simulink model "multiple_models_replacement"  (R2016a)
settings: Solver=VariableStepAuto  StartTime=0.0  StopTime=10.0  RelTol=1e-3
undefined symbols (not defined in the file): a2, b, b1, b2, eta, freq, g, J1, Jm1, Jw, Kem, kem, Kix, Kiy, Kpphi, Kpx, Kpy, kt, Kti, Kvphi, L, M, mi, mic, mis, N, R, r1, sigma0, sigma1, sigma2, Vdi, vs
settings Model: MinMaxOverflowLogging=ForceOff  sldv_blockreplacement_configurable_lib=multiple_models_rt_lib  Creator=Pichau  LastModifiedBy=Pichau
settings DataIOCC: SaveFormat=StructureWithTime  SaveOutput=off  SaveTime=off
settings DebuggingCC: ArtificialAlgebraicLoopMsg=none  SaveWithParameterizedLinksMsg=none  InheritedTsInSrcMsg=none  BusObjectLabelMismatch=none

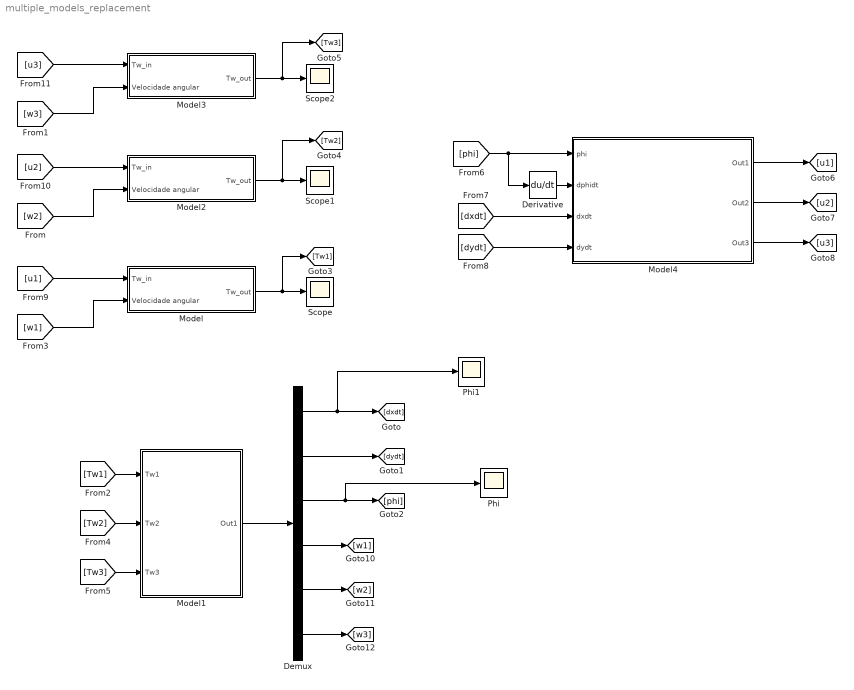
== system multiple_models_replacement ==
  Demux : Demux  Outputs=6
  Derivative : Derivative
  Model : Subsystem  TreatAsAtomicUnit=on  mask(Sldv ModelReference(Model name:modelo_eletrico) Replacement){ModelName=modelo_eletrico, ParameterArgumentNames=, ParameterArgumentValues=, SimulationMode=Normal}
      mask help: Replacement for the Model Reference block that references the model modelo_eletrico. If Model arguments are specified on the Model Reference block, then they will appear in the mask parameters.
  Model1 : Subsystem  TreatAsAtomicUnit=on  mask(Sldv ModelReference(Model name:modelo_mecanico) Replacement){ModelName=modelo_mecanico, ParameterArgumentNames=, ParameterArgumentValues=, SimulationMode=Normal}
      mask help: Replacement for the Model Reference block that references the model modelo_mecanico. If Model arguments are specified on the Model Reference block, then they will appear in the mask parameters.
  Model2 : Subsystem  TreatAsAtomicUnit=on  mask(Sldv ModelReference(Model name:modelo_eletrico) Replacement){ModelName=modelo_eletrico, ParameterArgumentNames=, ParameterArgumentValues=, SimulationMode=Normal}
      mask help: Replacement for the Model Reference block that references the model modelo_eletrico. If Model arguments are specified on the Model Reference block, then they will appear in the mask parameters.
  Model3 : Subsystem  TreatAsAtomicUnit=on  mask(Sldv ModelReference(Model name:modelo_eletrico) Replacement){ModelName=modelo_eletrico, ParameterArgumentNames=, ParameterArgumentValues=, SimulationMode=Normal}
      mask help: Replacement for the Model Reference block that references the model modelo_eletrico. If Model arguments are specified on the Model Reference block, then they will appear in the mask parameters.
  Model4 : Subsystem  TreatAsAtomicUnit=on  mask(Sldv ModelReference(Model name:resolved_acceleration_controller) Replacement){ModelName=resolved_acceleration_controller, ParameterArgumentNames=, ParameterArgumentValues=, SimulationMode=Normal}
      mask help: Replacement for the Model Reference block that references the model resolved_acceleration_controller. If Model arguments are specified on the Model Reference block, then they will appear in the mask parameters.
  Phi : Scope
  Phi1 : Scope
  Scope : Scope
  Scope1 : Scope
  Scope2 : Scope
  wires:
  [u1] -> Model/1(Tw_in)
  Model/1(Tw_out) -> [Tw1], Scope/1
  Model1/1(Out1) -> Demux/1
  Demux/3 -> Phi/1, [phi]
  Demux/4 -> [w1]
  Demux/5 -> [w2]
  Demux/6 -> [w3]
  Demux/1 -> Phi1/1, [dxdt]
  Demux/2 -> [dydt]
  [w1] -> Model/2(Velocidade angular)
  [u2] -> Model2/1(Tw_in)
  [w2] -> Model2/2(Velocidade angular)
  [u3] -> Model3/1(Tw_in)
  [w3] -> Model3/2(Velocidade angular)
  Model2/1(Tw_out) -> [Tw2], Scope1/1
  Model3/1(Tw_out) -> [Tw3], Scope2/1
  [Tw1] -> Model1/1(Tw1)
  [Tw3] -> Model1/3(Tw3)
  [Tw2] -> Model1/2(Tw2)
  Derivative/1 -> Model4/2(dphidt)
  [phi] -> Derivative/1, Model4/1(phi)
  [dxdt] -> Model4/3(dxdt)
  [dydt] -> Model4/4(dydt)
  Model4/1(Out1) -> [u1]
  Model4/2(Out2) -> [u2]
  Model4/3(Out3) -> [u3]

== system multiple_models_replacement/Model ==
  Tw_in : Inport  OutDataTypeStr=double  PortDimensions=1  SampleTime=[0,0]
  Velocidade angular : Inport  Port=2  OutDataTypeStr=double  PortDimensions=1  SampleTime=[0,0]
  1/r1 : Gain  Gain=r1
  1/r2 : Gain  Gain=r1
  Constant : Constant  Value=6
  Constant1 : Constant  Value=0.3
  Constant2 : Constant  Value=0
  Constant3 : Constant  Value=0
  Convergir torque para pulso : Subsystem
  Derivative : Derivative
  Roda1 : Subsystem
  dydt1 : Scope
  Tw_out : Outport  OutDataTypeStr=double  PortDimensions=1  SampleTime=[0,0]
  wires:
  Constant3/1 -> Roda1/6(s1)
  Constant2/1 -> Roda1/3(deltaVd1)
  Constant1/1 -> Roda1/1(Vsat1)
  Constant/1 -> Roda1/2(Vd1)
  1/r2/1 -> Tw_out/1
  Roda1/3(F1_aparente) -> 1/r2/1
  1/r1/1 -> Roda1/5(vel_lin1_aparente)
  [A] -> 1/r1/1
  Derivative/1 -> Convergir torque para pulso/2(aceleracao_angular)
  Velocidade angular/1 -> Derivative/1, [A], Convergir torque para pulso/3(velocidade angular)
  Tw_in/1 -> Convergir torque para pulso/1(Tw)
  Convergir torque para pulso/1(delta) -> dydt1/1, Roda1/4(u1)

== system multiple_models_replacement/Model1 ==
  Tw1 : Inport  OutDataTypeStr=double  PortDimensions=1  SampleTime=[0,0]
  Tw2 : Inport  Port=2  OutDataTypeStr=double  PortDimensions=1  SampleTime=[0,0]
  Tw3 : Inport  Port=3  OutDataTypeStr=double  PortDimensions=1  SampleTime=[0,0]
  Mux3 : Mux  Inputs=3
  Robô Omnidirecional : S-Function  FunctionName=espaco_de_estados  Parameters=r,m,Jw,J,L  SFunctionDeploymentMode=off  EnableBusSupport=off  mask{r=0.072, m=1.71, Jw=8.1e-4, J=2.125, L=0.09}
      mask prompts: r "r (m)"; m "m (Kg)"; Jw "Jw (Kg*m^2)"; J "J (Kg*m^2)"; L "L (m)"
      mask Display: image(imread('Robot_omnidirectional_drive.png'));
  Out1 : Outport  OutDataTypeStr=double  PortDimensions=6  SampleTime=[0,0]
  wires:
  Robô Omnidirecional/1 -> Out1/1
  Tw1/1 -> Mux3/1
  Tw2/1 -> Mux3/2
  Tw3/1 -> Mux3/3
  Mux3/1 -> Robô Omnidirecional/1

== system multiple_models_replacement/Model2 ==
  Tw_in : Inport  OutDataTypeStr=double  PortDimensions=1  SampleTime=[0,0]
  Velocidade angular : Inport  Port=2  OutDataTypeStr=double  PortDimensions=1  SampleTime=[0,0]
  1/r1 : Gain  Gain=r1
  1/r2 : Gain  Gain=r1
  Constant : Constant  Value=6
  Constant1 : Constant  Value=0.3
  Constant2 : Constant  Value=0
  Constant3 : Constant  Value=0
  Convergir torque para pulso : Subsystem
  Derivative : Derivative
  Roda1 : Subsystem
  dydt1 : Scope
  Tw_out : Outport  OutDataTypeStr=double  PortDimensions=1  SampleTime=[0,0]
  wires:
  Constant3/1 -> Roda1/6(s1)
  Constant2/1 -> Roda1/3(deltaVd1)
  Constant1/1 -> Roda1/1(Vsat1)
  Constant/1 -> Roda1/2(Vd1)
  1/r2/1 -> Tw_out/1
  Roda1/3(F1_aparente) -> 1/r2/1
  1/r1/1 -> Roda1/5(vel_lin1_aparente)
  [A] -> 1/r1/1
  Derivative/1 -> Convergir torque para pulso/2(aceleracao_angular)
  Velocidade angular/1 -> Derivative/1, [A], Convergir torque para pulso/3(velocidade angular)
  Tw_in/1 -> Convergir torque para pulso/1(Tw)
  Convergir torque para pulso/1(delta) -> dydt1/1, Roda1/4(u1)

== system multiple_models_replacement/Model3 ==
  Tw_in : Inport  OutDataTypeStr=double  PortDimensions=1  SampleTime=[0,0]
  Velocidade angular : Inport  Port=2  OutDataTypeStr=double  PortDimensions=1  SampleTime=[0,0]
  1/r1 : Gain  Gain=r1
  1/r2 : Gain  Gain=r1
  Constant : Constant  Value=6
  Constant1 : Constant  Value=0.3
  Constant2 : Constant  Value=0
  Constant3 : Constant  Value=0
  Convergir torque para pulso : Subsystem
  Derivative : Derivative
  Roda1 : Subsystem
  dydt1 : Scope
  Tw_out : Outport  OutDataTypeStr=double  PortDimensions=1  SampleTime=[0,0]
  wires:
  Constant3/1 -> Roda1/6(s1)
  Constant2/1 -> Roda1/3(deltaVd1)
  Constant1/1 -> Roda1/1(Vsat1)
  Constant/1 -> Roda1/2(Vd1)
  1/r2/1 -> Tw_out/1
  Roda1/3(F1_aparente) -> 1/r2/1
  1/r1/1 -> Roda1/5(vel_lin1_aparente)
  [A] -> 1/r1/1
  Derivative/1 -> Convergir torque para pulso/2(aceleracao_angular)
  Velocidade angular/1 -> Derivative/1, [A], Convergir torque para pulso/3(velocidade angular)
  Tw_in/1 -> Convergir torque para pulso/1(Tw)
  Convergir torque para pulso/1(delta) -> dydt1/1, Roda1/4(u1)

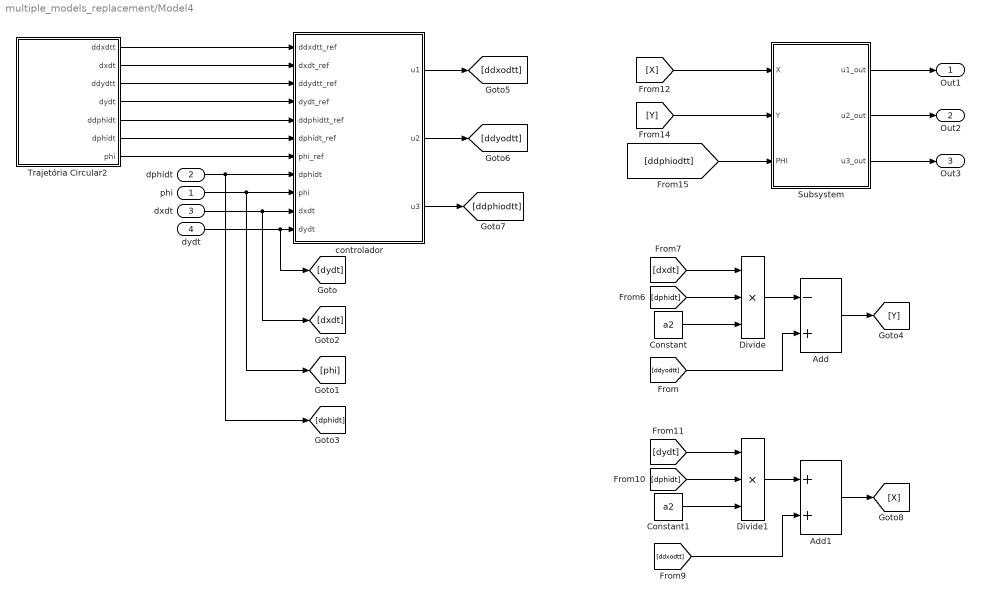
== system multiple_models_replacement/Model4 ==
  phi : Inport  OutDataTypeStr=double  PortDimensions=1  SampleTime=[0,0]
  dphidt : Inport  Port=2  OutDataTypeStr=double  PortDimensions=1  SampleTime=[0,0]
  dxdt : Inport  Port=3  OutDataTypeStr=double  PortDimensions=1  SampleTime=[0,0]
  dydt : Inport  Port=4  OutDataTypeStr=double  PortDimensions=1  SampleTime=[0,0]
  Add : Sum  Inputs=-+
  Add1 : Sum
  Constant : Constant  Value=a2
  Constant1 : Constant  Value=a2
  Divide : Product  Inputs=***
  Divide1 : Product  Inputs=***
  Subsystem : Subsystem
  Trajetória Circular2 : Subsystem
  controlador : Subsystem
  Out1 : Outport  OutDataTypeStr=double  PortDimensions=1  SampleTime=[0,0]
  Out2 : Outport  Port=2  OutDataTypeStr=double  PortDimensions=1  SampleTime=[0,0]
  Out3 : Outport  Port=3  OutDataTypeStr=double  PortDimensions=1  SampleTime=[0,0]
  wires:
  Subsystem/3(u3_out) -> Out3/1
  Subsystem/2(u2_out) -> Out2/1
  Subsystem/1(u1_out) -> Out1/1
  [ddphiodtt] -> Subsystem/3(PHI)
  [Y] -> Subsystem/2(Y)
  [X] -> Subsystem/1(X)
  Add1/1 -> [X]
  [ddxodtt] -> Add1/2
  Divide1/1 -> Add1/1
  [dydt] -> Divide1/1
  [dphidt] -> Divide1/2
  Constant1/1 -> Divide1/3
  Add/1 -> [Y]
  [ddyodtt] -> Add/2
  Divide/1 -> Add/1
  [dxdt] -> Divide/1
  [dphidt] -> Divide/2
  Constant/1 -> Divide/3
  dydt/1 -> [dydt], controlador/11(dydt)
  dxdt/1 -> [dxdt], controlador/10(dxdt)
  dphidt/1 -> [dphidt], controlador/8(dphidt)
  phi/1 -> [phi], controlador/9(phi)
  controlador/3(u3) -> [ddphiodtt]
  controlador/2(u2) -> [ddyodtt]
  controlador/1(u1) -> [ddxodtt]
  Trajetória Circular2/5(ddphidt) -> controlador/5(ddphidtt_ref)
  Trajetória Circular2/7(phi) -> controlador/7(phi_ref)
  Trajetória Circular2/3(ddydtt) -> controlador/3(ddydtt_ref)
  Trajetória Circular2/4(dydt) -> controlador/4(dydt_ref)
  Trajetória Circular2/1(ddxdtt) -> controlador/1(ddxdtt_ref)
  Trajetória Circular2/6(dphidt) -> controlador/6(dphidt_ref)
  Trajetória Circular2/2(dxdt) -> controlador/2(dxdt_ref)

== system multiple_models_replacement/Model/Convergir torque para pulso ==
  Tw : Inport
  aceleracao_angular : Inport  Port=2
  velocidade angular : Inport  Port=3
  Add : Sum  Inputs=+++
  Gain : Gain  Gain=R/(eta*N*Kti*Vdi)
  Gain1 : Gain  Gain=Kem
  Gain2 : Gain  Gain=R*Jw/(eta*N^2*Kti*Vdi)
  delta : Outport
  wires:
  aceleracao_angular/1 -> Gain2/1
  velocidade angular/1 -> Gain1/1
  Add/1 -> delta/1
  Tw/1 -> Gain/1
  Gain1/1 -> Add/3
  Gain/1 -> Add/1
  Gain2/1 -> Add/2

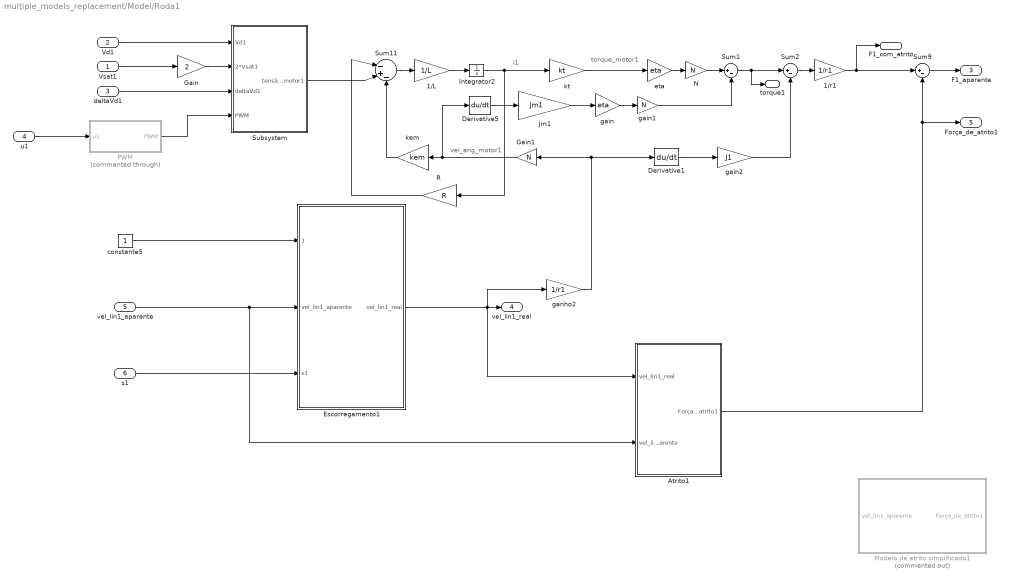
== system multiple_models_replacement/Model/Roda1 ==
  note: i1
  note: torque_motor1
  note: vel_ang_motor1
  Vsat1 : Inport
  Vd1 : Inport  Port=2
  deltaVd1 : Inport  Port=3
  u1 : Inport  Port=4
  vel_lin1_aparente : Inport  Port=5
  s1 : Inport  Port=6
  1/L : Gain  Gain=1/L
  1/r1 : Gain  Gain=1/r1
  Atrito1 : Subsystem
  Derivative1 : Derivative
  Derivative5 : Derivative
  Escorregamento1 : Subsystem
  Gain : Gain  Gain=2
  Gain1 : Gain  Gain=N
  Integrator2 : Integrator
  Jm1 : Gain  Gain=Jm1
  Modelo de atrito simplificado1 : Subsystem  Commented=on
  N : Gain  Gain=N
  PWM : Subsystem  Commented=through
  R : Gain  Gain=R
  Subsystem : Subsystem
  Sum1 : Sum  Inputs=|+-
  Sum11 : Sum  Inputs=|-+-
  Sum2 : Sum  Inputs=|+-
  Sum9 : Sum  Inputs=|+-
  constante5 : Constant
  eta : Gain  Gain=eta
  gain : Gain  Gain=eta
  gain1 : Gain  Gain=N
  gain2 : Gain  Gain=J1
  ganho2 : Gain  Gain=1/r1
  kem : Gain  Gain=kem
  kt : Gain  Gain=kt
  F1_com_atrito : Outport
  torque1 : Outport  Port=2
  F1_aparente : Outport  Port=3
  vel_lin1_real : Outport  Port=4
  Força_de_atrito1 : Outport  Port=5
  wires:
  Derivative5/1 -> Jm1/1
  Sum11/1 -> 1/L/1
  1/L/1 -> Integrator2/1
  Integrator2/1 -> kt/1, R/1
  Subsystem/1(tensão_motor1) -> Sum11/2
  kt/1 -> eta/1
  eta/1 -> N/1
  Gain1/1 -> kem/1, Derivative5/1
  1/r1/1 -> Sum9/1, F1_com_atrito/1
  Vsat1/1 -> Gain/1
  Vd1/1 -> Subsystem/1(Vd1)
  deltaVd1/1 -> Subsystem/3(deltaVd1)
  Gain/1 -> Subsystem/2("2*Vsat1 ")
  N/1 -> Sum1/1
  Sum1/1 -> torque1/1, Sum2/1
  gain/1 -> gain1/1
  Jm1/1 -> gain/1
  gain1/1 -> Sum1/2
  Derivative1/1 -> gain2/1
  gain2/1 -> Sum2/2
  Sum2/1 -> 1/r1/1
  kem/1 -> Sum11/3
  R/1 -> Sum11/1
  Sum9/1 -> F1_aparente/1
  u1/1 -> PWM/1(u1)
  Escorregamento1/1("vel_lin1_real ") -> Atrito1/1(vel_lin1_real), ganho2/1, vel_lin1_real/1
  ganho2/1 -> Derivative1/1, Gain1/1
  Atrito1/1(Força_de_atrito1) -> Sum9/2, Força_de_atrito1/1
  constante5/1 -> Escorregamento1/1(1)
  s1/1 -> Escorregamento1/3(s1)
  vel_lin1_aparente/1 -> Atrito1/2("vel_lin1_aparente "), Escorregamento1/2("vel_lin1_aparente ")
  PWM/1(PWM) -> Subsystem/4(PWM)

== system multiple_models_replacement/Model2/Convergir torque para pulso ==
  Tw : Inport
  aceleracao_angular : Inport  Port=2
  velocidade angular : Inport  Port=3
  Add : Sum  Inputs=+++
  Gain : Gain  Gain=R/(eta*N*Kti*Vdi)
  Gain1 : Gain  Gain=Kem
  Gain2 : Gain  Gain=R*Jw/(eta*N^2*Kti*Vdi)
  delta : Outport
  wires:
  aceleracao_angular/1 -> Gain2/1
  velocidade angular/1 -> Gain1/1
  Add/1 -> delta/1
  Tw/1 -> Gain/1
  Gain1/1 -> Add/3
  Gain/1 -> Add/1
  Gain2/1 -> Add/2

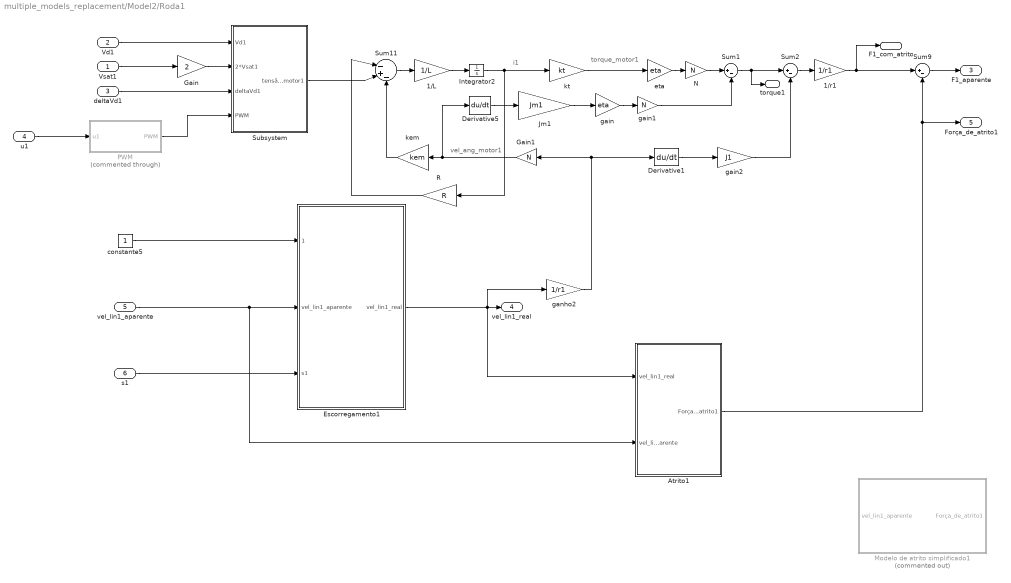
== system multiple_models_replacement/Model2/Roda1 ==
  note: i1
  note: torque_motor1
  note: vel_ang_motor1
  Vsat1 : Inport
  Vd1 : Inport  Port=2
  deltaVd1 : Inport  Port=3
  u1 : Inport  Port=4
  vel_lin1_aparente : Inport  Port=5
  s1 : Inport  Port=6
  1/L : Gain  Gain=1/L
  1/r1 : Gain  Gain=1/r1
  Atrito1 : Subsystem
  Derivative1 : Derivative
  Derivative5 : Derivative
  Escorregamento1 : Subsystem
  Gain : Gain  Gain=2
  Gain1 : Gain  Gain=N
  Integrator2 : Integrator
  Jm1 : Gain  Gain=Jm1
  Modelo de atrito simplificado1 : Subsystem  Commented=on
  N : Gain  Gain=N
  PWM : Subsystem  Commented=through
  R : Gain  Gain=R
  Subsystem : Subsystem
  Sum1 : Sum  Inputs=|+-
  Sum11 : Sum  Inputs=|-+-
  Sum2 : Sum  Inputs=|+-
  Sum9 : Sum  Inputs=|+-
  constante5 : Constant
  eta : Gain  Gain=eta
  gain : Gain  Gain=eta
  gain1 : Gain  Gain=N
  gain2 : Gain  Gain=J1
  ganho2 : Gain  Gain=1/r1
  kem : Gain  Gain=kem
  kt : Gain  Gain=kt
  F1_com_atrito : Outport
  torque1 : Outport  Port=2
  F1_aparente : Outport  Port=3
  vel_lin1_real : Outport  Port=4
  Força_de_atrito1 : Outport  Port=5
  wires:
  Derivative5/1 -> Jm1/1
  Sum11/1 -> 1/L/1
  1/L/1 -> Integrator2/1
  Integrator2/1 -> kt/1, R/1
  Subsystem/1(tensão_motor1) -> Sum11/2
  kt/1 -> eta/1
  eta/1 -> N/1
  Gain1/1 -> kem/1, Derivative5/1
  1/r1/1 -> Sum9/1, F1_com_atrito/1
  Vsat1/1 -> Gain/1
  Vd1/1 -> Subsystem/1(Vd1)
  deltaVd1/1 -> Subsystem/3(deltaVd1)
  Gain/1 -> Subsystem/2("2*Vsat1 ")
  N/1 -> Sum1/1
  Sum1/1 -> torque1/1, Sum2/1
  gain/1 -> gain1/1
  Jm1/1 -> gain/1
  gain1/1 -> Sum1/2
  Derivative1/1 -> gain2/1
  gain2/1 -> Sum2/2
  Sum2/1 -> 1/r1/1
  kem/1 -> Sum11/3
  R/1 -> Sum11/1
  Sum9/1 -> F1_aparente/1
  u1/1 -> PWM/1(u1)
  Escorregamento1/1("vel_lin1_real ") -> Atrito1/1(vel_lin1_real), ganho2/1, vel_lin1_real/1
  ganho2/1 -> Derivative1/1, Gain1/1
  Atrito1/1(Força_de_atrito1) -> Sum9/2, Força_de_atrito1/1
  constante5/1 -> Escorregamento1/1(1)
  s1/1 -> Escorregamento1/3(s1)
  vel_lin1_aparente/1 -> Atrito1/2("vel_lin1_aparente "), Escorregamento1/2("vel_lin1_aparente ")
  PWM/1(PWM) -> Subsystem/4(PWM)

== system multiple_models_replacement/Model3/Convergir torque para pulso ==
  Tw : Inport
  aceleracao_angular : Inport  Port=2
  velocidade angular : Inport  Port=3
  Add : Sum  Inputs=+++
  Gain : Gain  Gain=R/(eta*N*Kti*Vdi)
  Gain1 : Gain  Gain=Kem
  Gain2 : Gain  Gain=R*Jw/(eta*N^2*Kti*Vdi)
  delta : Outport
  wires:
  aceleracao_angular/1 -> Gain2/1
  velocidade angular/1 -> Gain1/1
  Add/1 -> delta/1
  Tw/1 -> Gain/1
  Gain1/1 -> Add/3
  Gain/1 -> Add/1
  Gain2/1 -> Add/2

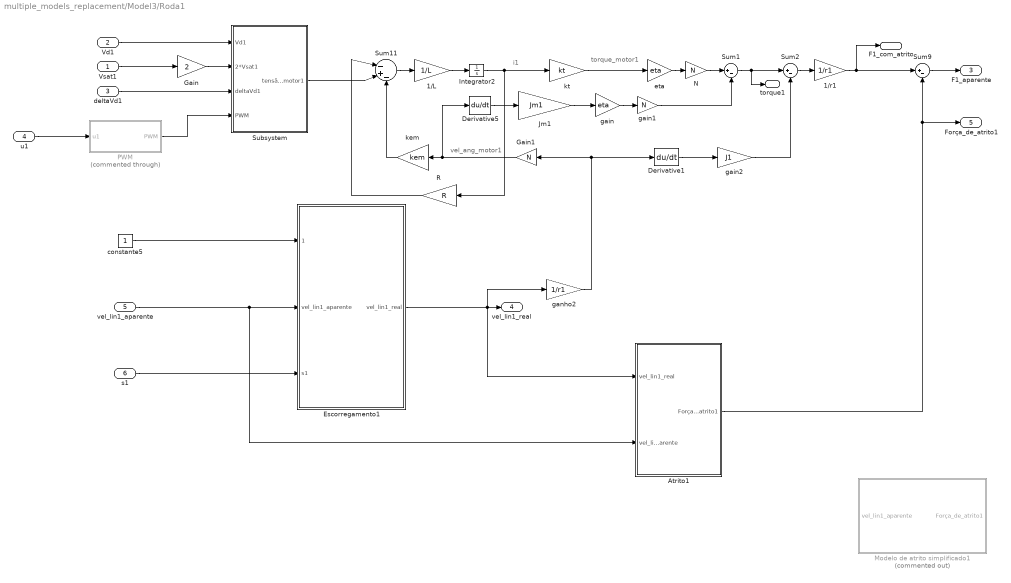
== system multiple_models_replacement/Model3/Roda1 ==
  note: i1
  note: torque_motor1
  note: vel_ang_motor1
  Vsat1 : Inport
  Vd1 : Inport  Port=2
  deltaVd1 : Inport  Port=3
  u1 : Inport  Port=4
  vel_lin1_aparente : Inport  Port=5
  s1 : Inport  Port=6
  1/L : Gain  Gain=1/L
  1/r1 : Gain  Gain=1/r1
  Atrito1 : Subsystem
  Derivative1 : Derivative
  Derivative5 : Derivative
  Escorregamento1 : Subsystem
  Gain : Gain  Gain=2
  Gain1 : Gain  Gain=N
  Integrator2 : Integrator
  Jm1 : Gain  Gain=Jm1
  Modelo de atrito simplificado1 : Subsystem  Commented=on
  N : Gain  Gain=N
  PWM : Subsystem  Commented=through
  R : Gain  Gain=R
  Subsystem : Subsystem
  Sum1 : Sum  Inputs=|+-
  Sum11 : Sum  Inputs=|-+-
  Sum2 : Sum  Inputs=|+-
  Sum9 : Sum  Inputs=|+-
  constante5 : Constant
  eta : Gain  Gain=eta
  gain : Gain  Gain=eta
  gain1 : Gain  Gain=N
  gain2 : Gain  Gain=J1
  ganho2 : Gain  Gain=1/r1
  kem : Gain  Gain=kem
  kt : Gain  Gain=kt
  F1_com_atrito : Outport
  torque1 : Outport  Port=2
  F1_aparente : Outport  Port=3
  vel_lin1_real : Outport  Port=4
  Força_de_atrito1 : Outport  Port=5
  wires:
  Derivative5/1 -> Jm1/1
  Sum11/1 -> 1/L/1
  1/L/1 -> Integrator2/1
  Integrator2/1 -> kt/1, R/1
  Subsystem/1(tensão_motor1) -> Sum11/2
  kt/1 -> eta/1
  eta/1 -> N/1
  Gain1/1 -> kem/1, Derivative5/1
  1/r1/1 -> Sum9/1, F1_com_atrito/1
  Vsat1/1 -> Gain/1
  Vd1/1 -> Subsystem/1(Vd1)
  deltaVd1/1 -> Subsystem/3(deltaVd1)
  Gain/1 -> Subsystem/2("2*Vsat1 ")
  N/1 -> Sum1/1
  Sum1/1 -> torque1/1, Sum2/1
  gain/1 -> gain1/1
  Jm1/1 -> gain/1
  gain1/1 -> Sum1/2
  Derivative1/1 -> gain2/1
  gain2/1 -> Sum2/2
  Sum2/1 -> 1/r1/1
  kem/1 -> Sum11/3
  R/1 -> Sum11/1
  Sum9/1 -> F1_aparente/1
  u1/1 -> PWM/1(u1)
  Escorregamento1/1("vel_lin1_real ") -> Atrito1/1(vel_lin1_real), ganho2/1, vel_lin1_real/1
  ganho2/1 -> Derivative1/1, Gain1/1
  Atrito1/1(Força_de_atrito1) -> Sum9/2, Força_de_atrito1/1
  constante5/1 -> Escorregamento1/1(1)
  s1/1 -> Escorregamento1/3(s1)
  vel_lin1_aparente/1 -> Atrito1/2("vel_lin1_aparente "), Escorregamento1/2("vel_lin1_aparente ")
  PWM/1(PWM) -> Subsystem/4(PWM)

== system multiple_models_replacement/Model4/Subsystem ==
  X : Inport
  Y : Inport  Port=2
  PHI : Inport  Port=3
  u1 : Subsystem
  u2 : Subsystem
  u3 : Subsystem
  u1_out : Outport
  u2_out : Outport  Port=2
  u3_out : Outport  Port=3
  wires:
  Y/1 -> u3/2(In2), u2/2(In2), u1/2(In2)
  PHI/1 -> u3/3(In3), u2/3(In3), u1/3(In3)
  X/1 -> u3/1(In1), u2/1(In1), u1/1(In1)
  u1/1(u1) -> u1_out/1
  u3/1(u3) -> u3_out/1
  u2/1(u2) -> u2_out/1

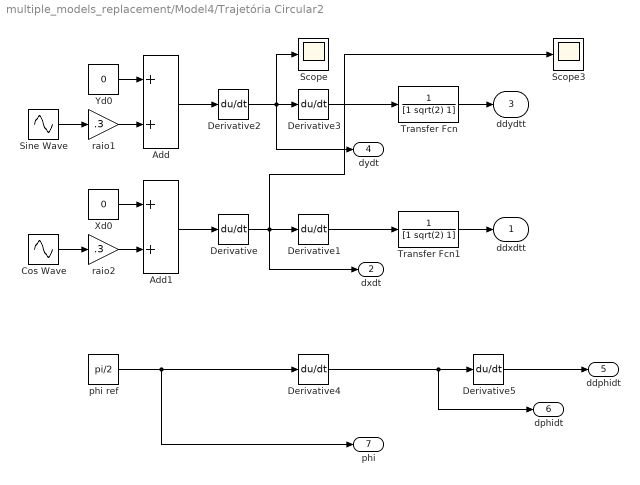
== system multiple_models_replacement/Model4/Trajetória Circular2 ==
  Add : Sum
  Add1 : Sum
  Cos Wave : Sin  Frequency=0.3  Phase=pi/2  SampleTime=0
  Derivative{,1..5} (6 alike) : Derivative
  Scope : Scope
  Scope3 : Scope
  Sine Wave : Sin  Frequency=0.3  SampleTime=0
  Transfer Fcn : TransferFcn  Denominator=[1 sqrt(2) 1]
  Transfer Fcn1 : TransferFcn  Denominator=[1 sqrt(2) 1]
  Xd0 : Constant  Value=0
  Yd0 : Constant  Value=0
  phi ref : Constant  Value=pi/2
  raio1 : Gain  Gain=.3
  raio2 : Gain  Gain=.3
  ddxdtt : Outport
  dxdt : Outport  Port=2
  ddydtt : Outport  Port=3
  dydt : Outport  Port=4
  ddphidt : Outport  Port=5
  dphidt : Outport  Port=6
  phi : Outport  Port=7
  wires:
  Transfer Fcn1/1 -> ddxdtt/1
  Transfer Fcn/1 -> ddydtt/1
  Derivative5/1 -> ddphidt/1
  Derivative1/1 -> Transfer Fcn1/1
  Derivative3/1 -> Transfer Fcn/1
  Derivative2/1 -> Derivative3/1, Scope/1, dydt/1
  Derivative/1 -> Scope3/1, Derivative1/1, dxdt/1
  Sine Wave/1 -> raio1/1
  raio1/1 -> Add/2
  Add/1 -> Derivative2/1
  Add1/1 -> Derivative/1
  raio2/1 -> Add1/2
  Cos Wave/1 -> raio2/1
  Xd0/1 -> Add1/1
  Yd0/1 -> Add/1
  phi ref/1 -> Derivative4/1, phi/1
  Derivative4/1 -> Derivative5/1, dphidt/1

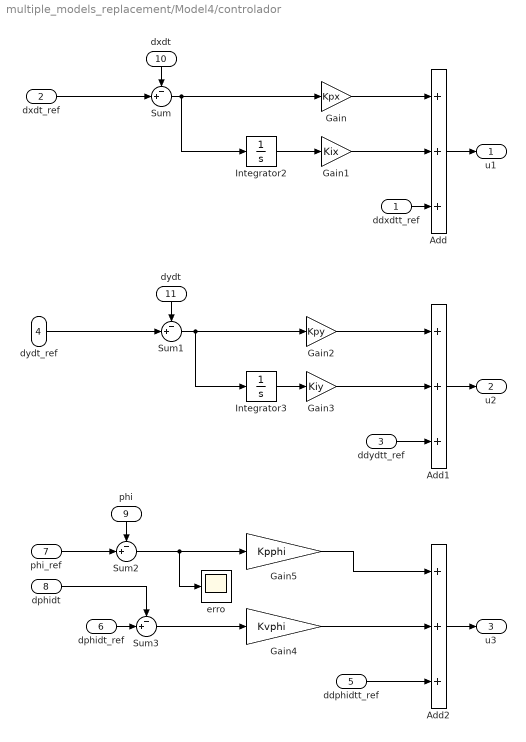
== system multiple_models_replacement/Model4/controlador ==
  ddxdtt_ref : Inport
  dxdt_ref : Inport  Port=2
  ddydtt_ref : Inport  Port=3
  dydt_ref : Inport  Port=4
  ddphidtt_ref : Inport  Port=5
  dphidt_ref : Inport  Port=6
  phi_ref : Inport  Port=7
  dphidt : Inport  Port=8
  phi : Inport  Port=9
  dxdt : Inport  Port=10
  dydt : Inport  Port=11
  Add : Sum  Inputs=+++
  Add1 : Sum  Inputs=+++
  Add2 : Sum  Inputs=+++
  Gain : Gain  Gain=Kpx
  Gain1 : Gain  Gain=Kix
  Gain2 : Gain  Gain=Kpy
  Gain3 : Gain  Gain=Kiy
  Gain4 : Gain  Gain=Kvphi
  Gain5 : Gain  Gain=Kpphi
  Integrator2 : Integrator
  Integrator3 : Integrator
  Sum{,1..3} (4 alike) : Sum  Inputs=-+|
  erro : Scope
  u1 : Outport
  u2 : Outport  Port=2
  u3 : Outport  Port=3
  wires:
  Sum2/1 -> Gain5/1, erro/1
  Sum1/1 -> Gain2/1, Integrator3/1
  Gain1/1 -> Add/2
  Integrator2/1 -> Gain1/1
  dydt_ref/1 -> Sum1/2
  Add/1 -> u1/1
  Gain2/1 -> Add1/1
  Integrator3/1 -> Gain3/1
  dphidt/1 -> Sum3/1
  Gain4/1 -> Add2/2
  Sum/1 -> Gain/1, Integrator2/1
  Gain3/1 -> Add1/2
  Gain5/1 -> Add2/1
  Sum3/1 -> Gain4/1
  ddphidtt_ref/1 -> Add2/3
  ddydtt_ref/1 -> Add1/3
  Add1/1 -> u2/1
  ddxdtt_ref/1 -> Add/3
  phi/1 -> Sum2/1
  Add2/1 -> u3/1
  dxdt_ref/1 -> Sum/2
  dxdt/1 -> Sum/1
  phi_ref/1 -> Sum2/2
  Gain/1 -> Add/1
  dydt/1 -> Sum1/1
  dphidt_ref/1 -> Sum3/2

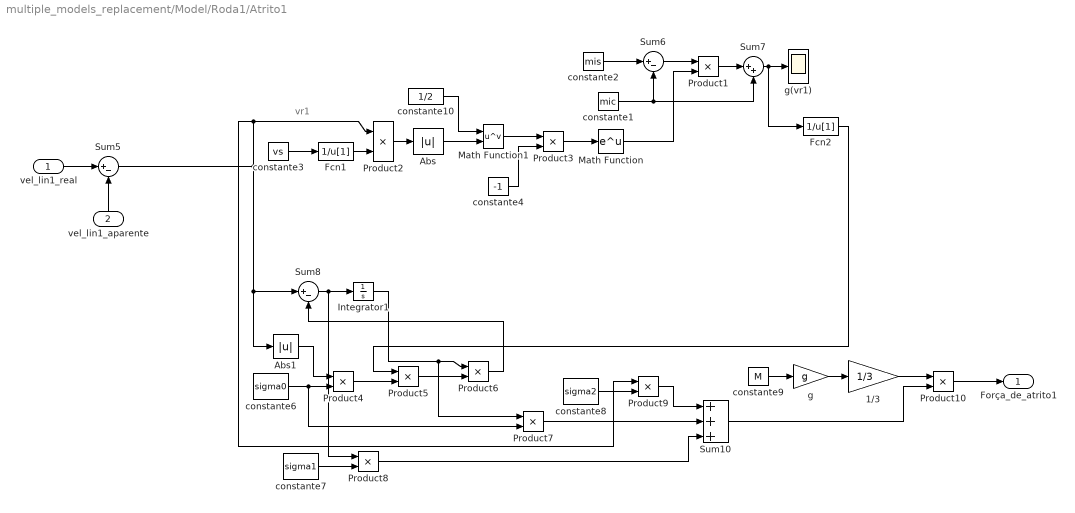
== system multiple_models_replacement/Model/Roda1/Atrito1 ==
  note: vr1
  vel_lin1_real : Inport
  "vel_lin1_aparente " : Inport  Port=2
  1/3 : Gain  Gain=1/3
  Abs : Abs
  Abs1 : Abs
  Fcn1 : Fcn  Expr=1/u[1]
  Fcn2 : Fcn  Expr=1/u[1]
  Integrator1 : Integrator
  Math Function : Math  SaturateOnIntegerOverflow=on
  Math Function1 : Math  Operator=pow  SaturateOnIntegerOverflow=on
  Product{1..10} (10 alike) : Product  RndMeth=Zero
  Sum10 : Sum  Inputs=+++
  Sum5 : Sum  Inputs=|+-
  Sum6 : Sum  Inputs=|+-
  Sum7 : Sum  Inputs=|++
  Sum8 : Sum  Inputs=|+-
  constante1 : Constant  Value=mic
  constante10 : Constant  Value=1/2
  constante2 : Constant  Value=mis
  constante3 : Constant  Value=vs
  constante4 : Constant  Value=-1
  constante6 : Constant  Value=sigma0
  constante7 : Constant  Value=sigma1
  constante8 : Constant  Value=sigma2
  constante9 : Constant  Value=M
  g : Gain  Gain=g
  g(vr1) : Scope
  Força_de_atrito1 : Outport
  wires:
  constante2/1 -> Sum6/1
  constante1/1 -> Sum6/2, Sum7/2
  Sum6/1 -> Product1/1
  constante3/1 -> Fcn1/1
  Fcn1/1 -> Product2/2
  Sum5/1 -> Sum8/1, Abs1/1, Product9/1, Product2/1
  Product2/1 -> Abs/1
  Abs/1 -> Math Function1/2
  Math Function1/1 -> Product3/1
  constante4/1 -> Product3/2
  Product3/1 -> Math Function/1
  Math Function/1 -> Product1/2
  Product1/1 -> Sum7/1
  Sum7/1 -> g(vr1)/1, Fcn2/1
  Sum8/1 -> Integrator1/1, Product8/1
  Integrator1/1 -> Product6/1, Product7/1
  constante6/1 -> Product4/2, Product7/2
  Abs1/1 -> Product4/1
  Product4/1 -> Product5/2
  Fcn2/1 -> Product5/1
  Product5/1 -> Product6/2
  Product6/1 -> Sum8/2
  constante7/1 -> Product8/2
  Product8/1 -> Sum10/3
  Product7/1 -> Sum10/2
  constante8/1 -> Product9/2
  Product9/1 -> Sum10/1
  constante9/1 -> g/1
  g/1 -> 1/3/1
  1/3/1 -> Product10/1
  Sum10/1 -> Product10/2
  constante10/1 -> Math Function1/1
  vel_lin1_real/1 -> Sum5/1
  "vel_lin1_aparente "/1 -> Sum5/2
  Product10/1 -> Força_de_atrito1/1

== system multiple_models_replacement/Model/Roda1/Escorregamento1 ==
  1 : Inport
  "vel_lin1_aparente " : Inport  Port=2
  s1 : Inport  Port=3
  Fcn : Fcn  Expr=1/u[1]
  Product : Product  RndMeth=Zero
  Sum3 : Sum  Inputs=+|+
  Sum4 : Sum  Inputs=|+-
  Switch : Switch
  "vel_lin1_real " : Outport
  wires:
  s1/1 -> Switch/2, Sum3/1, Sum4/2
  1/1 -> Sum3/2, Sum4/1
  Sum4/1 -> Fcn/1
  Fcn/1 -> Switch/1
  Sum3/1 -> Switch/3
  Switch/1 -> Product/2
  "vel_lin1_aparente "/1 -> Product/1
  Product/1 -> "vel_lin1_real "/1

== system multiple_models_replacement/Model/Roda1/Modelo de atrito simplificado1 ==
  vel_lin1_aparente : Inport
  1/3 : Gain  Gain=1/3
  Product10 : Product  RndMeth=Zero
  Scope : Scope
  Scope1 : Scope
  Scope2 : Scope
  Sign : Signum
  Sum1 : Sum  Inputs=++|
  Transfer Fcn : TransferFcn  Denominator=[0.001 1]
  constante9 : Constant  Value=M
  g : Gain  Gain=g
  g1 : Gain  Gain=mi
  g2 : Gain  Gain=b
  Força_de_atrito1 : Outport
  wires:
  Transfer Fcn/1 -> Força_de_atrito1/1, Scope2/1
  g2/1 -> Scope/1, Sum1/1
  Sum1/1 -> Transfer Fcn/1
  Sign/1 -> g1/1
  vel_lin1_aparente/1 -> Sign/1, g2/1
  Product10/1 -> Sum1/2, Scope1/1
  g1/1 -> Product10/2
  1/3/1 -> Product10/1
  g/1 -> 1/3/1
  constante9/1 -> g/1

== system multiple_models_replacement/Model/Roda1/PWM ==
  u1 : Inport
  Comparador : RelationalOperator  OutDataTypeStr=boolean
  Constant : Constant  Value=2
  Fcn : Fcn  Expr=2*(u(1)-0.5)
  Fcn1 : Fcn  Expr=2*((2*u[1]*freq)-0.5)
  Fcn2 : Fcn  Expr=u(1)-1
  Integrator : Integrator
  Onda Quadrada : Scope
  Onda Trinangular : Scope
  Product : Product  RndMeth=Zero
  Pulse Generator : DiscretePulseGenerator  PulseType=Time based  Period=1/freq  PulseWidth=50
  PWM : Outport
  wires:
  Pulse Generator/1 -> Fcn/1, Onda Quadrada/1
  Fcn/1 -> Integrator/1
  Integrator/1 -> Fcn1/1
  Fcn1/1 -> Onda Trinangular/1, Comparador/2
  u1/1 -> Comparador/1
  Fcn2/1 -> PWM/1
  Comparador/1 -> Product/2
  Product/1 -> Fcn2/1
  Constant/1 -> Product/1

== system multiple_models_replacement/Model/Roda1/Subsystem ==
  Vd1 : Inport
  "2*Vsat1 " : Inport  Port=2
  deltaVd1 : Inport  Port=3
  PWM : Inport  Port=4
  Product : Product  RndMeth=Zero
  Sum : Sum  Inputs=|+--
  tensão_motor1 : Outport
  wires:
  Sum/1 -> Product/1
  Vd1/1 -> Sum/1
  Product/1 -> tensão_motor1/1
  PWM/1 -> Product/2
  deltaVd1/1 -> Sum/3
  "2*Vsat1 "/1 -> Sum/2

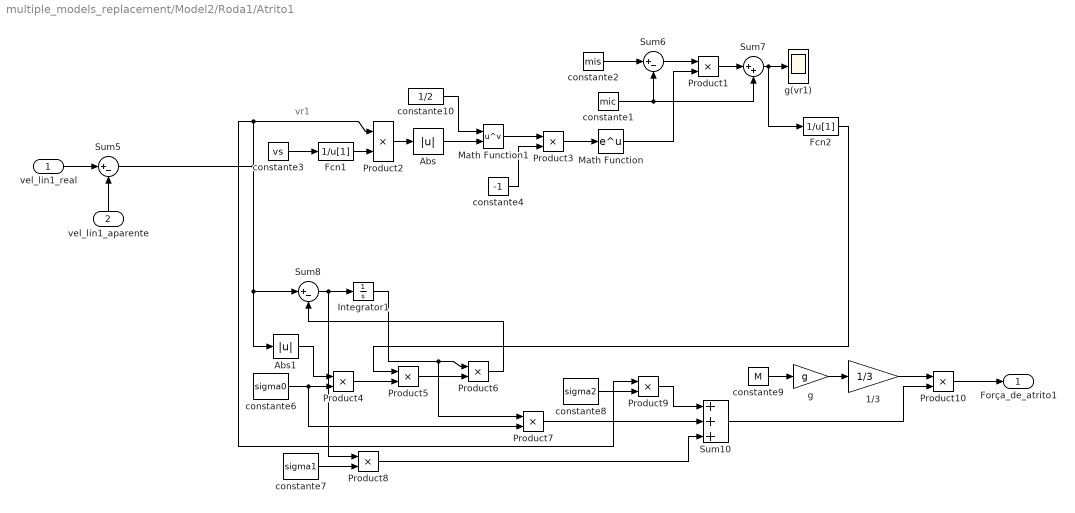
== system multiple_models_replacement/Model2/Roda1/Atrito1 ==
  note: vr1
  vel_lin1_real : Inport
  "vel_lin1_aparente " : Inport  Port=2
  1/3 : Gain  Gain=1/3
  Abs : Abs
  Abs1 : Abs
  Fcn1 : Fcn  Expr=1/u[1]
  Fcn2 : Fcn  Expr=1/u[1]
  Integrator1 : Integrator
  Math Function : Math  SaturateOnIntegerOverflow=on
  Math Function1 : Math  Operator=pow  SaturateOnIntegerOverflow=on
  Product{1..10} (10 alike) : Product  RndMeth=Zero
  Sum10 : Sum  Inputs=+++
  Sum5 : Sum  Inputs=|+-
  Sum6 : Sum  Inputs=|+-
  Sum7 : Sum  Inputs=|++
  Sum8 : Sum  Inputs=|+-
  constante1 : Constant  Value=mic
  constante10 : Constant  Value=1/2
  constante2 : Constant  Value=mis
  constante3 : Constant  Value=vs
  constante4 : Constant  Value=-1
  constante6 : Constant  Value=sigma0
  constante7 : Constant  Value=sigma1
  constante8 : Constant  Value=sigma2
  constante9 : Constant  Value=M
  g : Gain  Gain=g
  g(vr1) : Scope
  Força_de_atrito1 : Outport
  wires:
  constante2/1 -> Sum6/1
  constante1/1 -> Sum6/2, Sum7/2
  Sum6/1 -> Product1/1
  constante3/1 -> Fcn1/1
  Fcn1/1 -> Product2/2
  Sum5/1 -> Sum8/1, Abs1/1, Product9/1, Product2/1
  Product2/1 -> Abs/1
  Abs/1 -> Math Function1/2
  Math Function1/1 -> Product3/1
  constante4/1 -> Product3/2
  Product3/1 -> Math Function/1
  Math Function/1 -> Product1/2
  Product1/1 -> Sum7/1
  Sum7/1 -> g(vr1)/1, Fcn2/1
  Sum8/1 -> Integrator1/1, Product8/1
  Integrator1/1 -> Product6/1, Product7/1
  constante6/1 -> Product4/2, Product7/2
  Abs1/1 -> Product4/1
  Product4/1 -> Product5/2
  Fcn2/1 -> Product5/1
  Product5/1 -> Product6/2
  Product6/1 -> Sum8/2
  constante7/1 -> Product8/2
  Product8/1 -> Sum10/3
  Product7/1 -> Sum10/2
  constante8/1 -> Product9/2
  Product9/1 -> Sum10/1
  constante9/1 -> g/1
  g/1 -> 1/3/1
  1/3/1 -> Product10/1
  Sum10/1 -> Product10/2
  constante10/1 -> Math Function1/1
  vel_lin1_real/1 -> Sum5/1
  "vel_lin1_aparente "/1 -> Sum5/2
  Product10/1 -> Força_de_atrito1/1

== system multiple_models_replacement/Model2/Roda1/Escorregamento1 ==
  1 : Inport
  "vel_lin1_aparente " : Inport  Port=2
  s1 : Inport  Port=3
  Fcn : Fcn  Expr=1/u[1]
  Product : Product  RndMeth=Zero
  Sum3 : Sum  Inputs=+|+
  Sum4 : Sum  Inputs=|+-
  Switch : Switch
  "vel_lin1_real " : Outport
  wires:
  s1/1 -> Switch/2, Sum3/1, Sum4/2
  1/1 -> Sum3/2, Sum4/1
  Sum4/1 -> Fcn/1
  Fcn/1 -> Switch/1
  Sum3/1 -> Switch/3
  Switch/1 -> Product/2
  "vel_lin1_aparente "/1 -> Product/1
  Product/1 -> "vel_lin1_real "/1

== system multiple_models_replacement/Model2/Roda1/Modelo de atrito simplificado1 ==
  vel_lin1_aparente : Inport
  1/3 : Gain  Gain=1/3
  Product10 : Product  RndMeth=Zero
  Scope : Scope
  Scope1 : Scope
  Scope2 : Scope
  Sign : Signum
  Sum1 : Sum  Inputs=++|
  Transfer Fcn : TransferFcn  Denominator=[0.001 1]
  constante9 : Constant  Value=M
  g : Gain  Gain=g
  g1 : Gain  Gain=mi
  g2 : Gain  Gain=b
  Força_de_atrito1 : Outport
  wires:
  Transfer Fcn/1 -> Força_de_atrito1/1, Scope2/1
  g2/1 -> Scope/1, Sum1/1
  Sum1/1 -> Transfer Fcn/1
  Sign/1 -> g1/1
  vel_lin1_aparente/1 -> Sign/1, g2/1
  Product10/1 -> Sum1/2, Scope1/1
  g1/1 -> Product10/2
  1/3/1 -> Product10/1
  g/1 -> 1/3/1
  constante9/1 -> g/1

== system multiple_models_replacement/Model2/Roda1/PWM ==
  u1 : Inport
  Comparador : RelationalOperator  OutDataTypeStr=boolean
  Constant : Constant  Value=2
  Fcn : Fcn  Expr=2*(u(1)-0.5)
  Fcn1 : Fcn  Expr=2*((2*u[1]*freq)-0.5)
  Fcn2 : Fcn  Expr=u(1)-1
  Integrator : Integrator
  Onda Quadrada : Scope
  Onda Trinangular : Scope
  Product : Product  RndMeth=Zero
  Pulse Generator : DiscretePulseGenerator  PulseType=Time based  Period=1/freq  PulseWidth=50
  PWM : Outport
  wires:
  Pulse Generator/1 -> Fcn/1, Onda Quadrada/1
  Fcn/1 -> Integrator/1
  Integrator/1 -> Fcn1/1
  Fcn1/1 -> Onda Trinangular/1, Comparador/2
  u1/1 -> Comparador/1
  Fcn2/1 -> PWM/1
  Comparador/1 -> Product/2
  Product/1 -> Fcn2/1
  Constant/1 -> Product/1

== system multiple_models_replacement/Model2/Roda1/Subsystem ==
  Vd1 : Inport
  "2*Vsat1 " : Inport  Port=2
  deltaVd1 : Inport  Port=3
  PWM : Inport  Port=4
  Product : Product  RndMeth=Zero
  Sum : Sum  Inputs=|+--
  tensão_motor1 : Outport
  wires:
  Sum/1 -> Product/1
  Vd1/1 -> Sum/1
  Product/1 -> tensão_motor1/1
  PWM/1 -> Product/2
  deltaVd1/1 -> Sum/3
  "2*Vsat1 "/1 -> Sum/2

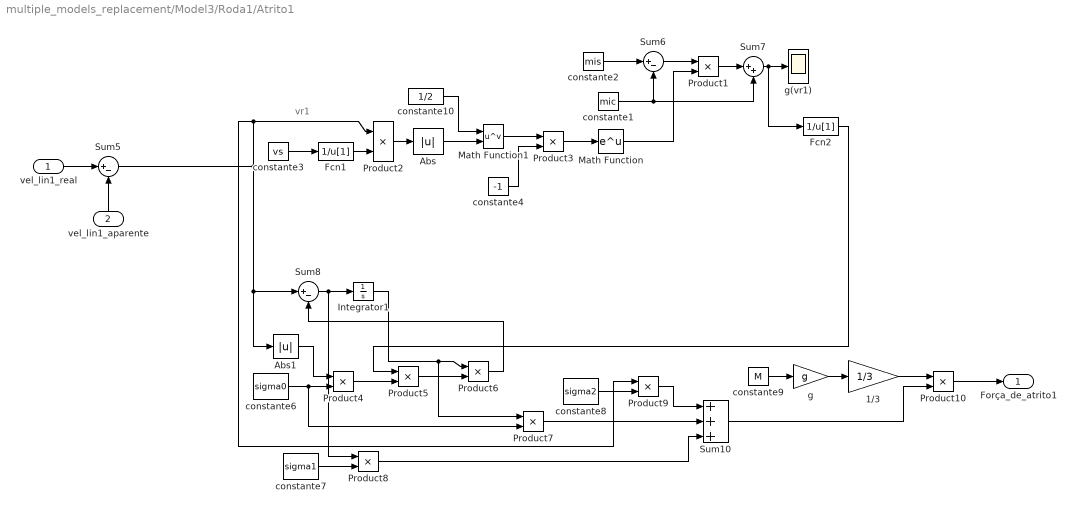
== system multiple_models_replacement/Model3/Roda1/Atrito1 ==
  note: vr1
  vel_lin1_real : Inport
  "vel_lin1_aparente " : Inport  Port=2
  1/3 : Gain  Gain=1/3
  Abs : Abs
  Abs1 : Abs
  Fcn1 : Fcn  Expr=1/u[1]
  Fcn2 : Fcn  Expr=1/u[1]
  Integrator1 : Integrator
  Math Function : Math  SaturateOnIntegerOverflow=on
  Math Function1 : Math  Operator=pow  SaturateOnIntegerOverflow=on
  Product{1..10} (10 alike) : Product  RndMeth=Zero
  Sum10 : Sum  Inputs=+++
  Sum5 : Sum  Inputs=|+-
  Sum6 : Sum  Inputs=|+-
  Sum7 : Sum  Inputs=|++
  Sum8 : Sum  Inputs=|+-
  constante1 : Constant  Value=mic
  constante10 : Constant  Value=1/2
  constante2 : Constant  Value=mis
  constante3 : Constant  Value=vs
  constante4 : Constant  Value=-1
  constante6 : Constant  Value=sigma0
  constante7 : Constant  Value=sigma1
  constante8 : Constant  Value=sigma2
  constante9 : Constant  Value=M
  g : Gain  Gain=g
  g(vr1) : Scope
  Força_de_atrito1 : Outport
  wires:
  constante2/1 -> Sum6/1
  constante1/1 -> Sum6/2, Sum7/2
  Sum6/1 -> Product1/1
  constante3/1 -> Fcn1/1
  Fcn1/1 -> Product2/2
  Sum5/1 -> Sum8/1, Abs1/1, Product9/1, Product2/1
  Product2/1 -> Abs/1
  Abs/1 -> Math Function1/2
  Math Function1/1 -> Product3/1
  constante4/1 -> Product3/2
  Product3/1 -> Math Function/1
  Math Function/1 -> Product1/2
  Product1/1 -> Sum7/1
  Sum7/1 -> g(vr1)/1, Fcn2/1
  Sum8/1 -> Integrator1/1, Product8/1
  Integrator1/1 -> Product6/1, Product7/1
  constante6/1 -> Product4/2, Product7/2
  Abs1/1 -> Product4/1
  Product4/1 -> Product5/2
  Fcn2/1 -> Product5/1
  Product5/1 -> Product6/2
  Product6/1 -> Sum8/2
  constante7/1 -> Product8/2
  Product8/1 -> Sum10/3
  Product7/1 -> Sum10/2
  constante8/1 -> Product9/2
  Product9/1 -> Sum10/1
  constante9/1 -> g/1
  g/1 -> 1/3/1
  1/3/1 -> Product10/1
  Sum10/1 -> Product10/2
  constante10/1 -> Math Function1/1
  vel_lin1_real/1 -> Sum5/1
  "vel_lin1_aparente "/1 -> Sum5/2
  Product10/1 -> Força_de_atrito1/1

== system multiple_models_replacement/Model3/Roda1/Escorregamento1 ==
  1 : Inport
  "vel_lin1_aparente " : Inport  Port=2
  s1 : Inport  Port=3
  Fcn : Fcn  Expr=1/u[1]
  Product : Product  RndMeth=Zero
  Sum3 : Sum  Inputs=+|+
  Sum4 : Sum  Inputs=|+-
  Switch : Switch
  "vel_lin1_real " : Outport
  wires:
  s1/1 -> Switch/2, Sum3/1, Sum4/2
  1/1 -> Sum3/2, Sum4/1
  Sum4/1 -> Fcn/1
  Fcn/1 -> Switch/1
  Sum3/1 -> Switch/3
  Switch/1 -> Product/2
  "vel_lin1_aparente "/1 -> Product/1
  Product/1 -> "vel_lin1_real "/1

== system multiple_models_replacement/Model3/Roda1/Modelo de atrito simplificado1 ==
  vel_lin1_aparente : Inport
  1/3 : Gain  Gain=1/3
  Product10 : Product  RndMeth=Zero
  Scope : Scope
  Scope1 : Scope
  Scope2 : Scope
  Sign : Signum
  Sum1 : Sum  Inputs=++|
  Transfer Fcn : TransferFcn  Denominator=[0.001 1]
  constante9 : Constant  Value=M
  g : Gain  Gain=g
  g1 : Gain  Gain=mi
  g2 : Gain  Gain=b
  Força_de_atrito1 : Outport
  wires:
  Transfer Fcn/1 -> Força_de_atrito1/1, Scope2/1
  g2/1 -> Scope/1, Sum1/1
  Sum1/1 -> Transfer Fcn/1
  Sign/1 -> g1/1
  vel_lin1_aparente/1 -> Sign/1, g2/1
  Product10/1 -> Sum1/2, Scope1/1
  g1/1 -> Product10/2
  1/3/1 -> Product10/1
  g/1 -> 1/3/1
  constante9/1 -> g/1

== system multiple_models_replacement/Model3/Roda1/PWM ==
  u1 : Inport
  Comparador : RelationalOperator  OutDataTypeStr=boolean
  Constant : Constant  Value=2
  Fcn : Fcn  Expr=2*(u(1)-0.5)
  Fcn1 : Fcn  Expr=2*((2*u[1]*freq)-0.5)
  Fcn2 : Fcn  Expr=u(1)-1
  Integrator : Integrator
  Onda Quadrada : Scope
  Onda Trinangular : Scope
  Product : Product  RndMeth=Zero
  Pulse Generator : DiscretePulseGenerator  PulseType=Time based  Period=1/freq  PulseWidth=50
  PWM : Outport
  wires:
  Pulse Generator/1 -> Fcn/1, Onda Quadrada/1
  Fcn/1 -> Integrator/1
  Integrator/1 -> Fcn1/1
  Fcn1/1 -> Onda Trinangular/1, Comparador/2
  u1/1 -> Comparador/1
  Fcn2/1 -> PWM/1
  Comparador/1 -> Product/2
  Product/1 -> Fcn2/1
  Constant/1 -> Product/1

== system multiple_models_replacement/Model3/Roda1/Subsystem ==
  Vd1 : Inport
  "2*Vsat1 " : Inport  Port=2
  deltaVd1 : Inport  Port=3
  PWM : Inport  Port=4
  Product : Product  RndMeth=Zero
  Sum : Sum  Inputs=|+--
  tensão_motor1 : Outport
  wires:
  Sum/1 -> Product/1
  Vd1/1 -> Sum/1
  Product/1 -> tensão_motor1/1
  PWM/1 -> Product/2
  deltaVd1/1 -> Sum/3
  "2*Vsat1 "/1 -> Sum/2

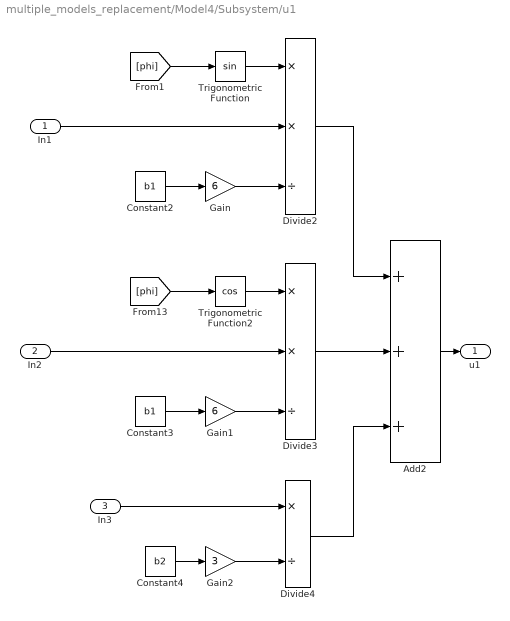
== system multiple_models_replacement/Model4/Subsystem/u1 ==
  In1 : Inport
  In2 : Inport  Port=2
  In3 : Inport  Port=3
  Add2 : Sum  Inputs=+++
  Constant2 : Constant  Value=b1
  Constant3 : Constant  Value=b1
  Constant4 : Constant  Value=b2
  Divide2 : Product  Inputs=**/
  Divide3 : Product  Inputs=**/
  Divide4 : Product  Inputs=*/
  Gain : Gain  Gain=6
  Gain1 : Gain  Gain=6
  Gain2 : Gain  Gain=3
  Trigonometric Function : Trigonometry
  Trigonometric Function2 : Trigonometry  Operator=cos
  u1 : Outport
  wires:
  Add2/1 -> u1/1
  Divide3/1 -> Add2/2
  Divide4/1 -> Add2/3
  In1/1 -> Divide2/2
  Gain2/1 -> Divide4/2
  Constant2/1 -> Gain/1
  Gain/1 -> Divide2/3
  [phi] -> Trigonometric Function/1
  Divide2/1 -> Add2/1
  Constant4/1 -> Gain2/1
  [phi] -> Trigonometric Function2/1
  Trigonometric Function2/1 -> Divide3/1
  In2/1 -> Divide3/2
  Constant3/1 -> Gain1/1
  Gain1/1 -> Divide3/3
  Trigonometric Function/1 -> Divide2/1
  In3/1 -> Divide4/1

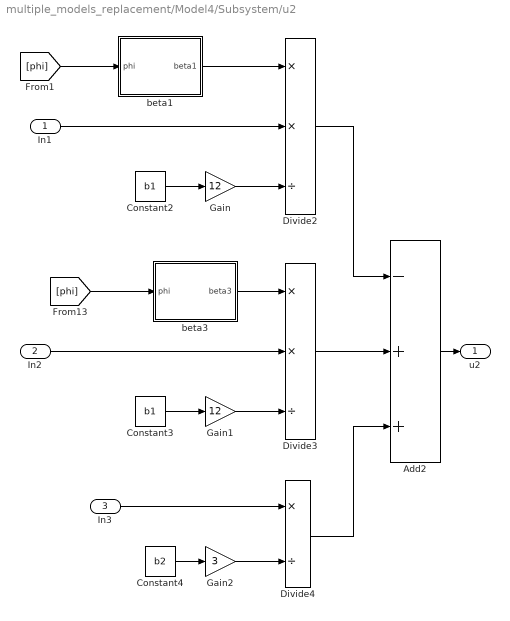
== system multiple_models_replacement/Model4/Subsystem/u2 ==
  In1 : Inport
  In2 : Inport  Port=2
  In3 : Inport  Port=3
  Add2 : Sum  Inputs=-++
  Constant2 : Constant  Value=b1
  Constant3 : Constant  Value=b1
  Constant4 : Constant  Value=b2
  Divide2 : Product  Inputs=**/
  Divide3 : Product  Inputs=**/
  Divide4 : Product  Inputs=*/
  Gain : Gain  Gain=12
  Gain1 : Gain  Gain=12
  Gain2 : Gain  Gain=3
  beta1 : Subsystem
  beta3 : Subsystem
  u2 : Outport
  wires:
  In3/1 -> Divide4/1
  beta1/1(beta1) -> Divide2/1
  Gain1/1 -> Divide3/3
  Constant3/1 -> Gain1/1
  In2/1 -> Divide3/2
  beta3/1(beta3) -> Divide3/1
  [phi] -> beta3/1(phi)
  Constant4/1 -> Gain2/1
  Divide2/1 -> Add2/1
  [phi] -> beta1/1(phi)
  Gain/1 -> Divide2/3
  Constant2/1 -> Gain/1
  Gain2/1 -> Divide4/2
  In1/1 -> Divide2/2
  Divide4/1 -> Add2/3
  Divide3/1 -> Add2/2
  Add2/1 -> u2/1

== system multiple_models_replacement/Model4/Subsystem/u3 ==
  In1 : Inport
  In2 : Inport  Port=2
  In3 : Inport  Port=3
  Add2 : Sum  Inputs=-++
  Constant2 : Constant  Value=b1
  Constant3 : Constant  Value=b1
  Constant4 : Constant  Value=b2
  Divide2 : Product  Inputs=**/
  Divide3 : Product  Inputs=**/
  Divide4 : Product  Inputs=*/
  Gain : Gain  Gain=12
  Gain1 : Gain  Gain=12
  Gain2 : Gain  Gain=3
  beta2 : Subsystem
  beta4 : Subsystem
  u3 : Outport
  wires:
  In3/1 -> Divide4/1
  beta2/1(beta2) -> Divide2/1
  Gain1/1 -> Divide3/3
  Constant3/1 -> Gain1/1
  In2/1 -> Divide3/2
  beta4/1(beta4) -> Divide3/1
  [phi] -> beta4/1(phi)
  Constant4/1 -> Gain2/1
  Divide2/1 -> Add2/1
  [phi] -> beta2/1(phi)
  Gain/1 -> Divide2/3
  Constant2/1 -> Gain/1
  Gain2/1 -> Divide4/2
  In1/1 -> Divide2/2
  Divide4/1 -> Add2/3
  Divide3/1 -> Add2/2
  Add2/1 -> u3/1

== system multiple_models_replacement/Model4/Subsystem/u2/beta1 ==
  phi : Inport
  Add2 : Sum  Inputs=+-
  Constant2 : Constant  Value=3
  Divide2 : Product  Inputs=**
  Sqrt : Sqrt  SaturateOnIntegerOverflow=on
  Trigonometric Function1 : Trigonometry  Operator=cos
  Trigonometric Function2 : Trigonometry
  beta1 : Outport
  wires:
  Trigonometric Function2/1 -> Add2/1
  phi/1 -> Trigonometric Function1/1, Trigonometric Function2/1
  Constant2/1 -> Sqrt/1
  Sqrt/1 -> Divide2/2
  Add2/1 -> beta1/1
  Trigonometric Function1/1 -> Divide2/1
  Divide2/1 -> Add2/2

== system multiple_models_replacement/Model4/Subsystem/u2/beta3 ==
  phi : Inport
  Add2 : Sum
  Constant2 : Constant  Value=3
  Divide2 : Product  Inputs=**
  Sqrt : Sqrt  SaturateOnIntegerOverflow=on
  Trigonometric Function1 : Trigonometry
  Trigonometric Function2 : Trigonometry  Operator=cos
  beta3 : Outport
  wires:
  Trigonometric Function2/1 -> Add2/1
  phi/1 -> Trigonometric Function1/1, Trigonometric Function2/1
  Constant2/1 -> Sqrt/1
  Sqrt/1 -> Divide2/2
  Add2/1 -> beta3/1
  Trigonometric Function1/1 -> Divide2/1
  Divide2/1 -> Add2/2

== system multiple_models_replacement/Model4/Subsystem/u3/beta2 ==
  phi : Inport
  Add2 : Sum
  Constant2 : Constant  Value=3
  Divide2 : Product  Inputs=**
  Sqrt : Sqrt  SaturateOnIntegerOverflow=on
  Trigonometric Function1 : Trigonometry  Operator=cos
  Trigonometric Function2 : Trigonometry
  beta2 : Outport
  wires:
  Divide2/1 -> Add2/2
  Trigonometric Function1/1 -> Divide2/1
  Add2/1 -> beta2/1
  Sqrt/1 -> Divide2/2
  Constant2/1 -> Sqrt/1
  phi/1 -> Trigonometric Function2/1, Trigonometric Function1/1
  Trigonometric Function2/1 -> Add2/1

== system multiple_models_replacement/Model4/Subsystem/u3/beta4 ==
  phi : Inport
  Add2 : Sum  Inputs=+-
  Constant2 : Constant  Value=3
  Divide2 : Product  Inputs=**
  Sqrt : Sqrt  SaturateOnIntegerOverflow=on
  Trigonometric Function1 : Trigonometry
  Trigonometric Function2 : Trigonometry  Operator=cos
  beta4 : Outport
  wires:
  Divide2/1 -> Add2/2
  Trigonometric Function1/1 -> Divide2/1
  Add2/1 -> beta4/1
  Sqrt/1 -> Divide2/2
  Constant2/1 -> Sqrt/1
  phi/1 -> Trigonometric Function2/1, Trigonometric Function1/1
  Trigonometric Function2/1 -> Add2/1
